simulink model "current"  (R2026a)
settings: Solver=FixedStepDiscrete  FixedStep=foc.Ts
PreLoadFcn:
  | try, p = fileparts(which(bdroot)); addpath(fullfile(p,'..', 'scripts')); addpath(fullfile(p,'..', 'models')); addpath(p); catch, end; init;
InitFcn:
  | try, p = fileparts(which(bdroot)); addpath(fullfile(p,'..', 'scripts')); addpath(fullfile(p,'..', 'models')); addpath(p); catch, end; init;
undefined symbols (not defined in the file): foc, pmsm
libraries: mcbeeMathTransformLib x3, slpidlib x2, mcbcontrolslib x2, mcbcontrollergainlib x1, mcbpositiondecoderlib x1
settings Model: Creator=probst  LastModifiedBy=niklasprobst
settings DebuggingCC: ParameterPrecisionLossMsg=none
settings HardwareCC: ProdLargestAtomicInteger=Integer  ProdHWDeviceType=Infineon->TriCore  TargetBitPerLong=64.0  TargetBitPerPointer=64.0  TargetBitPerSizeT=64.0  TargetBitPerPtrDiffT=64.0  TargetLongLongMode=on  TargetIntDivRoundTo=Zero  TargetEndianess=LittleEndian  TargetWordSize=64.0  TargetHWDeviceType=Custom Processor->MATLAB Host Computer  ProdEqTarget=off
settings RTWCC: SystemTargetFile=ert.tlc  Description=Embedded Coder
settings ERTTargetCC: GenerateSampleERTMain=on
settings SimscapeCC: SimscapeLogType=none

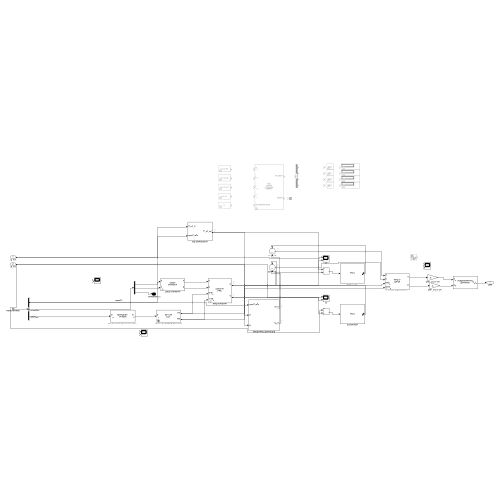
[thumbnail: Simulink's stored preview of the top-level diagram]
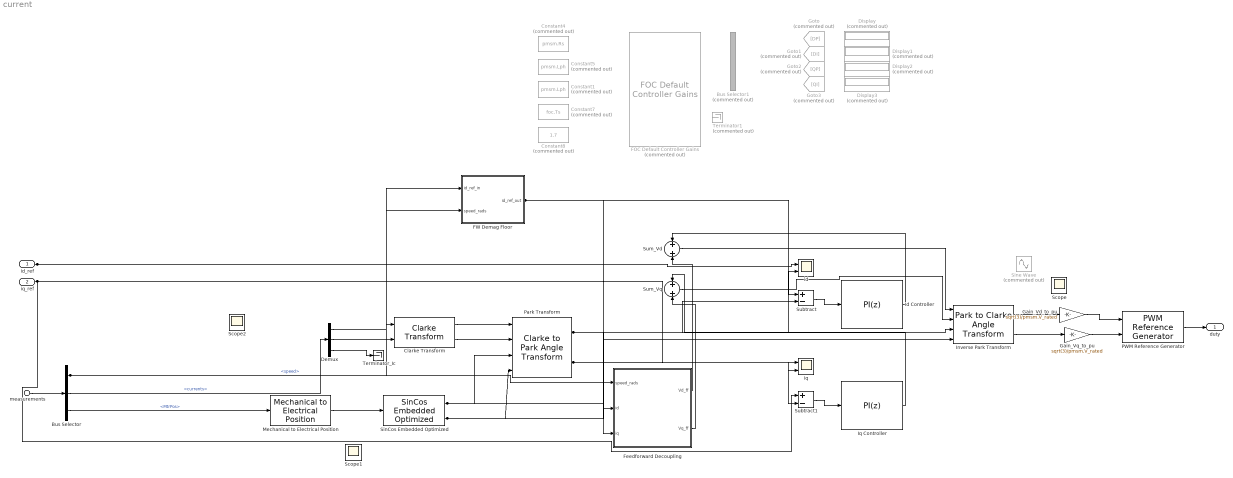
== system current ==
  id_ref : Inport
  iq_ref : Inport  Port=2
  measurements : Inport  Port=3  OutDataTypeStr=Bus: measurement
  Bus Selector : BusSelector  OutputSignals=speed,currents,MtrPos
  Bus Selector1 : BusSelector  Commented=on  OutputSignals=Daxis_Kp,Daxis_Ki*Ts,Qaxis_Kp,Qaxis_Ki*Ts
  Clarke Transform : mcbeeMathTransformLib/Clarke Transform  VariantControl=Variant2  PowerInvariant=off  UseWithEmbedded=on  PhaseInput=Two inputs
      settings: LibrarySourceBlock=mcblib/Controls/Math Transforms/Clarke Transform
  Constant1 : Constant  Commented=on  Value=pmsm.Lph
  Constant4 : Constant  Commented=on  Value=pmsm.Rs
  Constant5 : Constant  Commented=on  Value=pmsm.Lph
  Constant7 : Constant  Commented=on  Value=foc.Ts
  Constant8 : Constant  Commented=on  Value=1.7
  Demux : Demux  Outputs=[1 1 1]
  Display{,1..3} (4 alike) : Display  Commented=on
  FOC Default Controller Gains : mcbcontrollergainlib/FOC Default Controller Gains  Commented=on  ControllerGainType=Empirical method  motorSelection=PMSM  unitType=SI Unit  EnObserver=off  ObsType=Flux Observer (Only for SPMSM)  ObsCutOffFrq=10  outCurrentControlGain=on  outFWCGain=off  outSpeedControlGain=off  externalDelay=off  currentSensorDelay=50e-6  speedSensorDelay=50e-6  speedFilterDelay=0.02
  FW Demag Floor : Subsystem
  Feedforward Decoupling : Subsystem
  Gain_Vd_to_pu : Gain  Gain=sqrt(3)/pmsm.V_rated
  Gain_Vq_to_pu : Gain  Gain=sqrt(3)/pmsm.V_rated
  Goto : Goto  Commented=on  GotoTag=DP
  Goto1 : Goto  Commented=on  GotoTag=DI
  Goto2 : Goto  Commented=on  GotoTag=QP
  Goto3 : Goto  Commented=on  GotoTag=QI
  Id Controller : slpidlib/PID Controller  Controller=PI  Form=Parallel  TimeDomain=Discrete-time  UseExternalTs=off  SampleTime=foc.Ts  IntegratorMethod=Forward Euler  FilterMethod=Forward Euler  ControllerParametersSource=internal  P=foc.Kp_d  I=foc.Ki_d_Ts  UseKiTs=on  D=0  UseExternalDerivativeSource=off  N=100  UseFilter=on  TunerSelectOption=Transfer Function Based (PID Tuner App)  InitialConditionSource=internal  InitialConditionForIntegrator=0  InitialConditionForFilter=0  DifferentiatorICPrevScaledInput=0  ExternalReset=none  TrackingMode=off  Kt=1  LimitOutput=on  SatLimitsSource=internal  UpperSaturationLimit=foc.V_phase_max  LowerSaturationLimit=-foc.V_phase_max  LinearizeAsGain=on  AntiWindupMode=clamping  Kb=0.56841  LimitIntegrator=on  UpperIntegratorSaturationLimit=foc.V_phase_max  LowerIntegratorSaturationLimit=-foc.V_phase_max  RndMeth=Simplest  POutMin=[]  POutMax=[]  IOutMin=[]  IOutMax=[]  DOutMin=[]  DOutMax=[]  NOutMin=[]  NOutMax=[]  SumOutMin=[]  SumOutMax=[]  SaturationOutDataTypeStr=Inherit: Inherit via back propagation  SaturationOutMin=[]  SaturationOutMax=[]  PParamMin=[]  PParamMax=[]  IParamMin=[]  IParamMax=[]  DParamMin=[]  DParamMax=[]  NParamMin=[]  NParamMax=[]  KbParamMin=[]  KbParamMax=[]  KtParamMin=[]  KtParamMax=[]  KbOutMin=[]  KbOutMax=[]  KtOutMin=[]  KtOutMax=[]  IntegratorOutMin=[]  IntegratorOutMax=[]  FilterOutMin=[]  FilterOutMax=[]  SumI1OutMin=[]  SumI1OutMax=[]  SumI2OutMin=[]  SumI2OutMax=[]  SumI3OutMin=[]  SumI3OutMax=[]  SumI4OutMin=[]  SumI4OutMax=[]  SumDOutMin=[]  SumDOutMax=[]  DifferentiatorOutMin=[]  DifferentiatorOutMax=[]  FilterDiffOutCoefMin=[]  FilterDiffOutCoefMax=[]  ReciprocalOutMin=[]  ReciprocalOutMax=[]  SumDenOutMin=[]  SumDenOutMax=[]  SumNumOutMin=[]  SumNumOutMax=[]  DivideOutMin=[]  DivideOutMax=[]  UdiffTsProdOutMin=[]  UdiffTsProdOutMax=[]  NTsProdOutMin=[]  NTsProdOutMax=[]  UintegralTsProdOutMin=[]  UintegralTsProdOutMax=[]  UngainTsProdOutMin=[]  UngainTsProdOutMax=[]  ClampingZeroOutDataTypeStr=Inherit: Inherit via back propagation  ClampingZeroOutMin=[]  ClampingZeroOutMax=[]  FilterDenConstantOutDataTypeStr=Inherit: Inherit via back propagation  FilterDenConstantOutMin=[]  FilterDenConstantOutMax=[]  PCopyOutDataTypeStr=Inherit: Inherit via back propagation  PCopyOutMin=[]  PCopyOutMax=[]  NCopyOutDataTypeStr=Inherit: Inherit via back propagation  NCopyOutMin=[]  NCopyOutMax=[]  IntegratorContinuousStateAttributes=''  IntegratorStateMustResolveToSignalObject=off  IntegratorRTWStateStorageClass=Auto  FilterContinuousStateAttributes=''  FilterStateMustResolveToSignalObject=off  FilterRTWStateStorageClass=Auto  ParallelPVariant=InternalParameters  IdealPVariant=Disabled  IVariant=InternalParameters  DVariant=Disabled  IntegratorVariant=Discrete  SatVariant=Enabled  AWVariant=DiscClampingParallel  PCopyVariant=Disabled  TRVariant=Disabled  FdbkBlocksVariant=Forward  IdealPFdbkVariant=Disabled  SatFdbkVariant=Disabled  DerivativeFilterVariant=Disabled  NVariant=Disabled  NCopyVariant=Disabled_SignalSpec  FilterICVariant=Disabled  IntegratorICVariant=InternalICs  ExternalResetVariant=Disabled  TRSumVariant=Passthrough  SumFdbkVariant=Disabled  SumVariant=Sum_PI  TsampFilterVariant=InternalTs  TsampNgainVariant=Passthrough  TsampIntegralVariant=Disabled_SignalSpec  ExternalSaturationOutDataTypeStr=Inherit: Same as second input  DerivativeSourceVariant=Disabled  PreIntVariant=InternalPreInt
      settings: LibrarySourceBlock=mcblib/Controls/Controllers/PI Controller
  Inverse Park Transform : mcbeeMathTransformLib/Park to Clarke Angle Transform  AxisAlignment=D-axis  UseWithEmbedded=on  PhaseInput=Two inputs  ThetaInput=Sine and Cosine electrical position  AngleInput=Per-unit  N_points=1024
      settings: LibrarySourceBlock=mcblib/Controls/Math Transforms/Inverse Park Transform
  Iq Controller : slpidlib/PID Controller  Controller=PI  Form=Parallel  TimeDomain=Discrete-time  UseExternalTs=off  SampleTime=foc.Ts  IntegratorMethod=Forward Euler  FilterMethod=Forward Euler  ControllerParametersSource=internal  P=foc.Kp_q  I=foc.Ki_q_Ts  UseKiTs=on  D=0  UseExternalDerivativeSource=off  N=100  UseFilter=on  TunerSelectOption=Transfer Function Based (PID Tuner App)  InitialConditionSource=internal  InitialConditionForIntegrator=0  InitialConditionForFilter=0  DifferentiatorICPrevScaledInput=0  ExternalReset=none  TrackingMode=off  Kt=1  LimitOutput=on  SatLimitsSource=internal  UpperSaturationLimit=foc.V_phase_max  LowerSaturationLimit=-foc.V_phase_max  LinearizeAsGain=on  AntiWindupMode=clamping  Kb=0.36172  LimitIntegrator=on  UpperIntegratorSaturationLimit=foc.V_phase_max  LowerIntegratorSaturationLimit=-foc.V_phase_max  RndMeth=Simplest  POutMin=[]  POutMax=[]  IOutMin=[]  IOutMax=[]  DOutMin=[]  DOutMax=[]  NOutMin=[]  NOutMax=[]  SumOutMin=[]  SumOutMax=[]  SaturationOutDataTypeStr=Inherit: Inherit via back propagation  SaturationOutMin=[]  SaturationOutMax=[]  PParamMin=[]  PParamMax=[]  IParamMin=[]  IParamMax=[]  DParamMin=[]  DParamMax=[]  NParamMin=[]  NParamMax=[]  KbParamMin=[]  KbParamMax=[]  KtParamMin=[]  KtParamMax=[]  KbOutMin=[]  KbOutMax=[]  KtOutMin=[]  KtOutMax=[]  IntegratorOutMin=[]  IntegratorOutMax=[]  FilterOutMin=[]  FilterOutMax=[]  SumI1OutMin=[]  SumI1OutMax=[]  SumI2OutMin=[]  SumI2OutMax=[]  SumI3OutMin=[]  SumI3OutMax=[]  SumI4OutMin=[]  SumI4OutMax=[]  SumDOutMin=[]  SumDOutMax=[]  DifferentiatorOutMin=[]  DifferentiatorOutMax=[]  FilterDiffOutCoefMin=[]  FilterDiffOutCoefMax=[]  ReciprocalOutMin=[]  ReciprocalOutMax=[]  SumDenOutMin=[]  SumDenOutMax=[]  SumNumOutMin=[]  SumNumOutMax=[]  DivideOutMin=[]  DivideOutMax=[]  UdiffTsProdOutMin=[]  UdiffTsProdOutMax=[]  NTsProdOutMin=[]  NTsProdOutMax=[]  UintegralTsProdOutMin=[]  UintegralTsProdOutMax=[]  UngainTsProdOutMin=[]  UngainTsProdOutMax=[]  ClampingZeroOutDataTypeStr=Inherit: Inherit via back propagation  ClampingZeroOutMin=[]  ClampingZeroOutMax=[]  FilterDenConstantOutDataTypeStr=Inherit: Inherit via back propagation  FilterDenConstantOutMin=[]  FilterDenConstantOutMax=[]  PCopyOutDataTypeStr=Inherit: Inherit via back propagation  PCopyOutMin=[]  PCopyOutMax=[]  NCopyOutDataTypeStr=Inherit: Inherit via back propagation  NCopyOutMin=[]  NCopyOutMax=[]  IntegratorContinuousStateAttributes=''  IntegratorStateMustResolveToSignalObject=off  IntegratorRTWStateStorageClass=Auto  FilterContinuousStateAttributes=''  FilterStateMustResolveToSignalObject=off  FilterRTWStateStorageClass=Auto  ParallelPVariant=InternalParameters  IdealPVariant=Disabled  IVariant=InternalParameters  DVariant=Disabled  IntegratorVariant=Discrete  SatVariant=Enabled  AWVariant=DiscClampingParallel  PCopyVariant=Disabled  TRVariant=Disabled  FdbkBlocksVariant=Forward  IdealPFdbkVariant=Disabled  SatFdbkVariant=Disabled  DerivativeFilterVariant=Disabled  NVariant=Disabled  NCopyVariant=Disabled_SignalSpec  FilterICVariant=Disabled  IntegratorICVariant=InternalICs  ExternalResetVariant=Disabled  TRSumVariant=Passthrough  SumFdbkVariant=Disabled  SumVariant=Sum_PI  TsampFilterVariant=InternalTs  TsampNgainVariant=Passthrough  TsampIntegralVariant=Disabled_SignalSpec  ExternalSaturationOutDataTypeStr=Inherit: Same as second input  DerivativeSourceVariant=Disabled  PreIntVariant=InternalPreInt
      settings: LibrarySourceBlock=mcblib/Controls/Controllers/PI Controller
  Mechanical to Electrical Position : mcbpositiondecoderlib/Mechanical to Electrical Position  PolePairsInputType=Specify via dialog  NrPP=pmsm.P  selectedRange=Radians  MechOfstInputType=Specify via dialog  mechOffsetIn=0  maxAngleIn=2*pi  InputDataType=single  VariantSelect=floating-point
      settings: LibrarySourceBlock=mcblib/Sensor Decoders/Mechanical to Electrical Position
  PWM Reference Generator : mcbcontrolslib/PWM Reference Generator  modType=SVM: space vector modulation  inSignal=Valphabeta  expandVoltageInput=on  inputUnits=Per-unit  LimitModulation=off  enableVoltage=off  enableModulationSignal=off  enableDutyCycle=on  expandVoltageOutput=on
      settings: LibrarySourceBlock=mcblib/Controls/Math Transforms/PWM Reference Generator
  Park Transform : mcbeeMathTransformLib/Clarke to Park Angle Transform  AxisAlignment=D-axis  UseWithEmbedded=on  PhaseInput=Two inputs  ThetaInput=Sine and Cosine electrical position  AngleInput=Per-unit  N_points=1024
      settings: LibrarySourceBlock=mcblib/Controls/Math Transforms/Park Transform
  Scope : Scope  NumInputPorts=2
      settings: ActiveDisplayYMinimum=-612.37163560148008  ActiveDisplayYMaximum=612.37189243028615
  Scope1 : Scope  NumInputPorts=2
      settings: ActiveDisplayYMinimum=-3.5597814582216527  ActiveDisplayYMaximum=6.3570651964002307  DataLoggingVariableName=ScopeData3
  Scope2 : Scope
      settings: ActiveDisplayYMinimum=-32.366468450824122  ActiveDisplayYMaximum=31.57884615980204  DataLoggingVariableName=ScopeData4
  SinCos Embedded Optimized : mcbcontrolslib/SinCos Embedded Optimized  LabelModeActiveChoice=MCB_Sin  OptforProc=off  OptLevelPop=Disabled  ApproximationMethod=None  UserApproxMethod=Lookup  ApproxStatus=None  ThetaDataType=single  CopyThetaDataType=single  InterpMethod=Linear point-slope  NumberOfDataPoints=16  NumberOfIterations=11  RemoveProtectionAgainstOutOfRangeInput=off  TableDataTypeStr=Inherit: Inherit via input  AngleInput=Radians  CopyAngleInput=Radians  N_points=1024  CopyN_points=1024  Datatype=Inherit: Same as input  CopyTableDatatype=Inherit: Same as input  DatatypeInput=Inherit from input  IsPrevStrictOpt=0  IsPrevLUTForced=0
      settings: LibrarySourceBlock=mcblib/Controls/Math Transforms/SinCos Embedded Optimized
  Sine Wave : Sin  Commented=on  Frequency=2*pi*100  Phase=[0, -pi/2]  SampleTime=0
  Subtract : Sum  Inputs=+-
  Subtract1 : Sum  Inputs=+-
  Sum_Vd : Sum
  Sum_Vq : Sum
  Terminator1 : Terminator  Commented=on
  Terminator_Ic : Terminator
  id : Scope  NumInputPorts=2
      settings: ActiveDisplayYMinimum=-11.362731179125216  ActiveDisplayYMaximum=12.204147478436571
  iq : Scope  NumInputPorts=2
      settings: ActiveDisplayYMinimum=-43.481506402956065  ActiveDisplayYMaximum=105.58190007147998  DataLoggingVariableName=ScopeData2
  duty : Outport
  wires:
  measurements/1 -> Bus Selector/1
  Bus Selector/2 -> Demux/1  "<currents>"
  Demux/1 -> Clarke Transform/1
  Demux/2 -> Clarke Transform/2
  Demux/3 -> Terminator_Ic/1
  Bus Selector/3 -> Mechanical to Electrical Position/1  "<MtrPos>"
  Mechanical to Electrical Position/1 -> SinCos Embedded Optimized/1
  Clarke Transform/1 -> Park Transform/1
  Clarke Transform/2 -> Park Transform/2
  SinCos Embedded Optimized/1 -> Park Transform/3, Inverse Park Transform/3
  SinCos Embedded Optimized/2 -> Park Transform/4, Inverse Park Transform/4
  id_ref/1 -> id/1, FW Demag Floor/1(id_ref_in)
  Park Transform/1 -> Subtract/2, id/2
  iq_ref/1 -> Subtract1/1, Feedforward Decoupling/3(iq), iq/1
  Park Transform/2 -> Subtract1/2, iq/2
  Subtract/1 -> Id Controller/1
  Subtract1/1 -> Iq Controller/1
  Bus Selector/1 -> Feedforward Decoupling/1(speed_rads), FW Demag Floor/2(speed_rads)  "<speed>"
  Id Controller/1 -> Sum_Vd/1
  Feedforward Decoupling/1(Vd_ff) -> Sum_Vd/2
  Iq Controller/1 -> Sum_Vq/1
  Feedforward Decoupling/2(Vq_ff) -> Sum_Vq/2
  Sum_Vd/1 -> Inverse Park Transform/1
  Sum_Vq/1 -> Inverse Park Transform/2
  Inverse Park Transform/1 -> Gain_Vd_to_pu/1
  Inverse Park Transform/2 -> Gain_Vq_to_pu/1
  Gain_Vd_to_pu/1 -> PWM Reference Generator/1
  Gain_Vq_to_pu/1 -> PWM Reference Generator/2
  PWM Reference Generator/1 -> duty/1
  FW Demag Floor/1(id_ref_out) -> Subtract/1, Feedforward Decoupling/2(id)

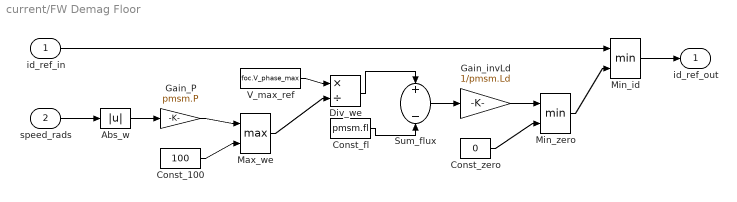
== system current/FW Demag Floor ==
  id_ref_in : Inport
  speed_rads : Inport  Port=2
  Abs_w : Abs  SaturateOnIntegerOverflow=off
  Const_100 : Constant  Value=100
  Const_fl : Constant  Value=pmsm.fl
  Const_zero : Constant  Value=0
  Div_we : Product  Inputs=*/
  Gain_P : Gain  Gain=pmsm.P
  Gain_invLd : Gain  Gain=1/pmsm.Ld
  Max_we : MinMax  Function=max  Inputs=2
  Min_id : MinMax  Inputs=2
  Min_zero : MinMax  Inputs=2
  Sum_flux : Sum  Inputs=+-
  V_max_ref : Constant  Value=foc.V_phase_max
  id_ref_out : Outport
  wires:
  ? -> ?
  speed_rads/1 -> Abs_w/1
  Abs_w/1 -> Gain_P/1
  Gain_P/1 -> Max_we/1
  Const_100/1 -> Max_we/2
  V_max_ref/1 -> Div_we/1
  Max_we/1 -> Div_we/2
  Div_we/1 -> Sum_flux/1
  Const_fl/1 -> Sum_flux/2
  Sum_flux/1 -> Gain_invLd/1
  Gain_invLd/1 -> Min_zero/1
  Const_zero/1 -> Min_zero/2
  id_ref_in/1 -> Min_id/1
  Min_zero/1 -> Min_id/2
  Min_id/1 -> id_ref_out/1

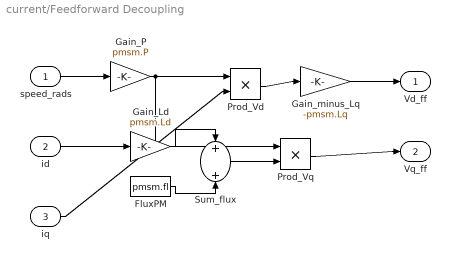
== system current/Feedforward Decoupling ==
  speed_rads : Inport
  id : Inport  Port=2
  iq : Inport  Port=3
  FluxPM : Constant  Value=pmsm.fl
  Gain_Ld : Gain  Gain=pmsm.Ld
  Gain_P : Gain  Gain=pmsm.P
  Gain_minus_Lq : Gain  Gain=-pmsm.Lq
  Prod_Vd : Product
  Prod_Vq : Product
  Sum_flux : Sum
  Vd_ff : Outport
  Vq_ff : Outport  Port=2
  wires:
  ? -> ?
  speed_rads/1 -> Gain_P/1
  Gain_P/1 -> Prod_Vd/1, Prod_Vq/1
  iq/1 -> Prod_Vd/2
  Prod_Vd/1 -> Gain_minus_Lq/1
  Gain_minus_Lq/1 -> Vd_ff/1
  id/1 -> Gain_Ld/1
  Gain_Ld/1 -> Sum_flux/1
  FluxPM/1 -> Sum_flux/2
  Sum_flux/1 -> Prod_Vq/2
  Prod_Vq/1 -> Vq_ff/1
